simulink model "sim_autom97"  (Simulink 6.2)
settings: Solver=ode45  StartTime=0.0  StopTime=Tmax  MaxStep=0.01*T  RelTol=1e-3
undefined symbols (not defined in the file or in its folder): dF, dK, dR, nF, nK, nR, T, tauF
settings Model: LastModifiedBy=Administrator
settings OptimizationCC: InlineInvariantSignals=on
settings HardwareCC: TargetUnknown=on

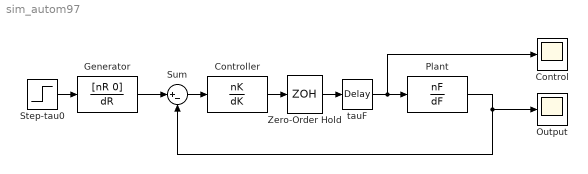
== system sim_autom97 ==
  Control : Scope
      settings: TimeRange=10  YMin=-50  YMax=50  SaveName=u  DataFormat=Array
  Controller : DiscreteTransferFcn  Numerator=nK  Denominator=dK  SampleTime=T
  Generator : TransferFcn  Numerator=[nR 0]  Denominator=dR
  Output : Scope
      settings: TimeRange=10  YMin=-4  YMax=6  SaveName=y  DataFormat=Array
  Plant : TransferFcn  Numerator=nF  Denominator=dF
  Step-tau0 : Step  Time=0
  Sum : Sum  Inputs=|+-  SaturateOnIntegerOverflow=on  InputSameDT=on
  Zero-Order Hold : ZeroOrderHold  SampleTime=T
  tauF : TransportDelay  DelayTime=tauF  BufferSize=10240
  wires:
  Step-tau0/1 -> Generator/1
  Controller/1 -> Zero-Order Hold/1
  Zero-Order Hold/1 -> tauF/1
  tauF/1 -> Plant/1, Control/1
  Sum/1 -> Controller/1
  Plant/1 -> Sum/2, Output/1
  Generator/1 -> Sum/1
